simulink library "SingleDofForceElement"  (Simulink 6.0)
settings: Solver=ode45  SolverMode=SingleTasking  StartTime=0.0  StopTime=10.0  RelTol=1e-3
libraries: mblibv1 x2
settings Model: Creator=vchudnov  LastModifiedBy=batserve  ExtModeAutoUpdateStatusClock=off
settings OptimizationCC: BooleanDataType=off
settings DebuggingCC: SolverPrmCheckMsg=none
settings HardwareCC: TargetUnknown=on

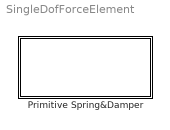
== system SingleDofForceElement ==
  Primitive Spring&Damper : Subsystem  AncestorBlock=SingleDofForceElement/Primitive Spring&Damper  mask{actuatedPrimitive=P1, springPositionOffset=0, damperVelocityOffset=0, springConstant=0, damperConstant=0, positionUnits=km, angleUnits=deg, velocityUnits=km/s, angleVelocityUnits=deg/s, forceUnits=N, torqueUnits=N-m}
      mask prompts: actuatedPrimitive "Primitive:"; springPositionOffset "Position Offset:"; damperVelocityOffset "Velocity Offset:"; springConstant "Spring Constant:"; damperConstant "Damping Constant:"; positionUnits "Linear Position Units:"; angleUnits "Angular Position Units:"; velocityUnits "Linear Velocity Units:"; angleVelocityUnits "Angular Velocity Units:"; forceUnits "Force Units:"; torqueUnits "Torque Units:"
      mask help:
      | A spring/damper element for a single degree of freedom. This subsystem implements a force relation of the type
      | F = -k*(x-x0) + -b*v, where k, b, and x are the spring constant, the damper constant, and the spring position offset, respectively.
      |
      | To set values for the spring/damper parameters, please click and open the Force Element block directly.
      mask init:
      | mech_primitivespringdamper;
      mask Help: To set values for the spring/damper parameters, please click and open the Force Element block directly.
      mask StyleString: popup(P1|P2|P3|R1|R2|R3),edit,edit,edit,edit,popup(km|m|cm|mm|mi|ft|in),popup(deg|rad),popup(km/s|m/s|cm/s|mm/s|mi/s|ft/s|in/s),popup(deg/s|rad/s),popup(N|lb),popup(N-m|ft-lb)

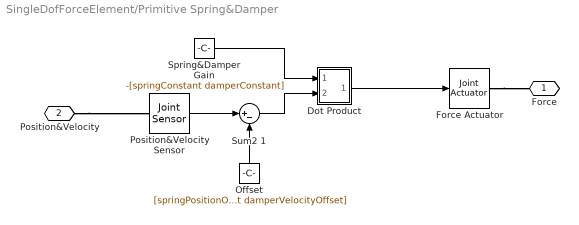
== system SingleDofForceElement/Primitive Spring&Damper ==
  Dot Product : Subsystem  AncestorBlock=simulink/Math Operations/Dot Product  mask(Dot Product){}
      mask help:
      | Inner (dot) product.
      | y = sum(conj(u1).*u2). The operand u1 corresponds to the top (or left) input port.
      mask init:
      | t=(0:.1:2*pi)';
      | x=cos(t);
      | y=sin(t);
      | r=0.05;
      mask Help: Computes the inner (dot) product of the inputs: sum(u1.*u2).  The inputs are vectors of the same length. Output is a scalar.
      mask Display: patch([x*r+0.5],[y*r+0.5])
  Force Actuator : mblibv1/Sensors &  Actuators/Joint Actuator  Tag=__orphan__  PortType=blob  PhysicalDomain=Mechanical  ActuationStyle=Force  AngleUnits=deg  ArcVelocityUnits=deg/s  ArcAccelerationUnits=deg/s^2  CoordPositionUnits=m  VelocityUnits=m/s  AccelerationUnits=m/s^2  ForceUnits=N  TorqueUnits=N-m  ActiveIO=off  Width=1  DialogClass=MechanicalActuatorBlock  Primitive=P1  ReferenceFrame=Absolute (INERTIAL)
  Offset : Constant  Orientation=up  Value=[springPositionOffset damperVelocityOffset]
  Position&Velocity Sensor : mblibv1/Sensors &  Actuators/Joint Sensor  Tag=__orphan__  PortType=blob  PhysicalDomain=Mechanical  Muxed=on  Pose=off  Angle=on  AngleUnits=deg  ArcVelocity=on  ArcVelocityUnits=deg/s  ArcAcceleration=off  ArcAccelerationUnits=deg/s^2  CoordPosition=on  CoordPositionUnits=km  Velocity=on  VelocityUnits=km/s  Acceleration=off  AccelerationUnits=m/s^2  Quaternion=off  QuaternionDT=off  QuaternionDDT=off  QuaternionUnits=deg  OutputVector=[ 1 1 1 1 ]  ActiveIO=off  Width=1  DialogClass=MechanicalSensorBlock  Primitive=P1  Force=off  ForceUnits=N  Torque=off  TorqueUnits=N-m  ReferenceFrame=Absolute (INERTIAL)  ReactionSensedSide=Base  ReactionReferenceFrame=Absolute (World)  ReactionForce=off  ReactionForceUnits=N  ReactionMoment=off  ReactionMomentUnits=N-m
  Spring&Damper Gain : Constant  Value=-[springConstant damperConstant]
  Sum2 1 : Sum  Inputs=|+-  SaturateOnIntegerOverflow=on
  Force : PMIOPort  Orientation=left  Port=1  Side=Right
  Position&Velocity : PMIOPort  Port=2  Side=Left
  wires:
  Position&Velocity Sensor/1 -> Sum2 1/1
  Offset/1 -> Sum2 1/2
  Dot Product/1(Out1) -> Force Actuator/1
  Sum2 1/1 -> Dot Product/2(In2)
  Spring&Damper Gain/1 -> Dot Product/1(In1)
  connections:
  Position&Velocity/RConn1 -- Position&Velocity Sensor/LConn1
  Force Actuator/RConn1 -- Force/RConn1

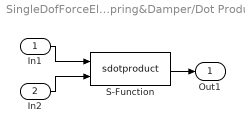
== system SingleDofForceElement/Primitive Spring&Damper/Dot Product ==
  In1 : Inport  Port=1  LatchInput=off
  In2 : Inport  Port=2  LatchInput=off
  S-Function : S-Function  FunctionName=sdotproduct
  Out1 : Outport
  wires:
  S-Function/1 -> Out1/1
  In1/1 -> S-Function/1
  In2/1 -> S-Function/2
